simulink model "buckConverterVCM"  (R2024a)
settings: Solver=VariableStepAuto  StartTime=0.0  StopTime=.2  MaxStep=.00001  RelTol=1e-3
model workspace (MAT data in the model file):
  C = Simulink.Parameter
  C.Value = 1e-05
  C.Complexity = 'real'
  C.Dimensions = [1 1]
  C.DataType = 'auto'
  L = Simulink.Parameter
  L.Value = 0.00022
  L.Complexity = 'real'
  L.Dimensions = [1 1]
  L.DataType = 'auto'
  R = Simulink.Parameter
  R.Value = 5
  R.Complexity = 'real'
  R.Dimensions = [1 1]
  R.DataType = 'auto'
  Vin = Simulink.Parameter
  Vin.Value = 48
  Vin.Complexity = 'real'
  Vin.Dimensions = [1 1]
  Vin.DataType = 'auto'
values from neighbouring files (symbols this model uses):
  Fs = 1e5    (= 100000)    [lineToOutputTF.m]
  H = Vref/Vin    (= 0.1)    [lineToOutputTF.m]
  L = 220*10^-6    (= 0.00022)    [lineToOutputTF.m]
  R = Vo/Io    (= 6)    [lineToOutputTF.m]
  R1 = 1e4    (= 10000)    [lineToOutputTF.m]
  R2 = 9e4    (= 90000)    [lineToOutputTF.m]
  Vin = 50    [lineToOutputTF.m]
  Vo = 12    [lineToOutputTF.m]
libraries: spsSeriesRLCBranchLib x5, spsCurrentMeasurementLib x2, spsVoltageMeasurementLib x2, spsControlledVoltageSourceLib x1, spsDiodeLib x1, spsMosfetLib x1, simulink x1, spspowerguiLib x1
settings Model: Creator=User  LastModifiedBy=User
settings DebuggingCC: UnconnectedInputMsg=warning  UnconnectedOutputMsg=warning  UnconnectedLineMsg=warning
settings ModelReferenceCC: EnableRefExpFcnMdlSchedulingChecks=on
settings RTWCC: GPUComputeCapability=3.5  DLArmComputeVersion=19.05

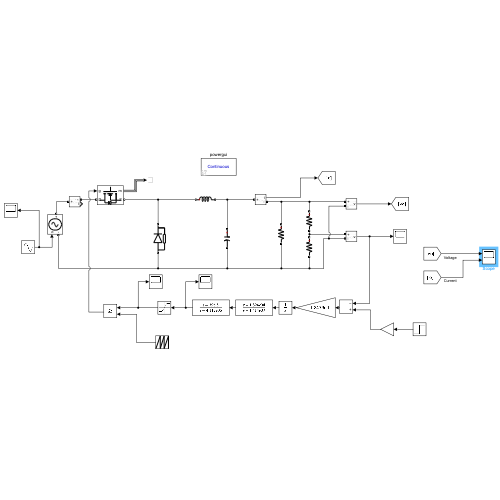
[thumbnail: Simulink's stored preview of the top-level diagram]
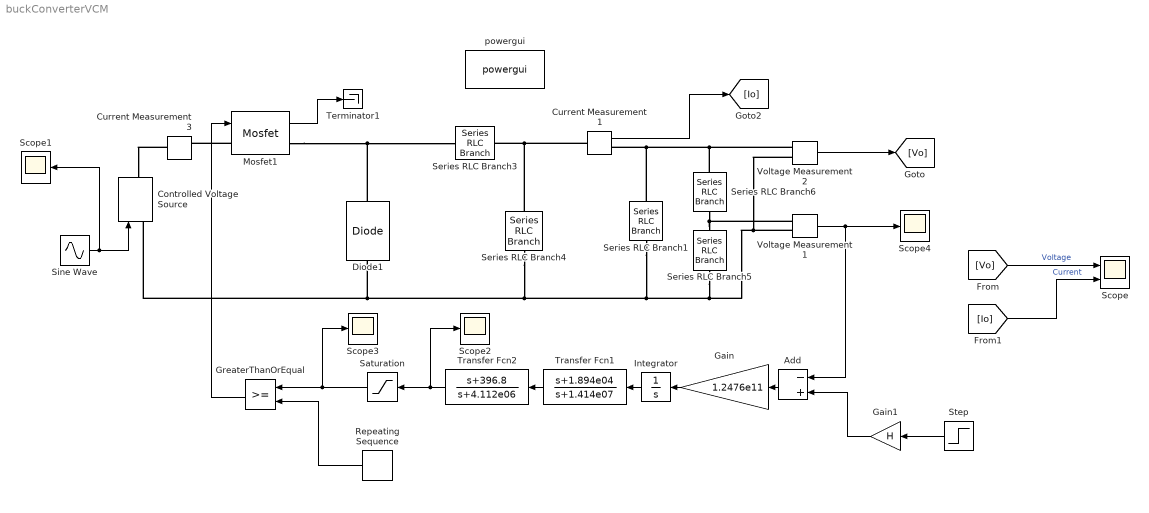
== system buckConverterVCM ==
  Add : Sum  Inputs=-+
  Controlled Voltage Source : spsControlledVoltageSourceLib/Controlled Voltage Source  Initialize=on  Source_Type=AC  Amplitude=0  Phase=0  Frequency=0  Measurements=None
  Current Measurement1 : spsCurrentMeasurementLib/Current Measurement  PhasorSimulation=off  OutputType=Complex  PSBequivalent=0
  Current Measurement3 : spsCurrentMeasurementLib/Current Measurement  PhasorSimulation=off  OutputType=Complex  PSBequivalent=0
  Diode1 : spsDiodeLib/Diode  Ron=0.001  Lon=0  Vf=0.8  IC=0  UseSnubber=0  Rs=500  Cs=250e-9  Measurements=off
  Gain : Gain  Gain=1.2476e11
  Gain1 : Gain  Gain=H
  GreaterThanOrEqual : RelationalOperator  OutDataTypeStr=boolean  RndMeth=Simplest  InputSameDT=off
  Integrator : Integrator
  Mosfet1 : spsMosfetLib/Mosfet  Ron=0.1  Lon=0  Rd=0.01  Vfd=0  IC=0  Rs=1e5  Cs=inf  Measurements=on
  Repeating Sequence : simulink/Sources/Repeating Sequence  rep_seq_t=[0 1]/Fs  rep_seq_y=[0 1]
  Saturation : Saturate  UpperLimit=.9  LowerLimit=.1
  Scope : Scope  NumInputPorts=2
  Scope{1..4} (4 alike) : Scope
  Series RLC Branch1 : spsSeriesRLCBranchLib/Series RLC Branch  LConnTagsString=__new0  RConnTagsString=__new0  BranchType=R  Resistance=R  Inductance=1e-3  SetiL0=off  InitialCurrent=0  Capacitance=1e-6  Setx0=off  InitialVoltage=0  Measurements=None
  Series RLC Branch3 : spsSeriesRLCBranchLib/Series RLC Branch  LConnTagsString=__new0  RConnTagsString=__new0  BranchType=L  Resistance=1  Inductance=L  SetiL0=off  InitialCurrent=0  Capacitance=1e-6  Setx0=off  InitialVoltage=0  Measurements=None
  Series RLC Branch4 : spsSeriesRLCBranchLib/Series RLC Branch  LConnTagsString=__new0  RConnTagsString=__new0  BranchType=C  Resistance=1  Inductance=1e-3  SetiL0=off  InitialCurrent=0  Capacitance=5*10^-4  Setx0=off  InitialVoltage=0  Measurements=None
  Series RLC Branch5 : spsSeriesRLCBranchLib/Series RLC Branch  LConnTagsString=__new0  RConnTagsString=__new0  BranchType=R  Resistance=R1  Inductance=1e-3  SetiL0=off  InitialCurrent=0  Capacitance=1e-6  Setx0=off  InitialVoltage=0  Measurements=None
  Series RLC Branch6 : spsSeriesRLCBranchLib/Series RLC Branch  LConnTagsString=__new0  RConnTagsString=__new0  BranchType=R  Resistance=R2  Inductance=1e-3  SetiL0=off  InitialCurrent=0  Capacitance=1e-6  Setx0=off  InitialVoltage=0  Measurements=None
  Sine Wave : Sin  Amplitude=2  Bias=Vin  Frequency=2*pi*100  SampleTime=0
  Step : Step  Time=0  After=Vo  SampleTime=0
  Terminator1 : Terminator
  Transfer Fcn1 : TransferFcn  Numerator=[1 1.894e04]  Denominator=[1 1.414e07]
  Transfer Fcn2 : TransferFcn  Numerator=[1 396.8]  Denominator=[1 4.112e06]
  Voltage Measurement1 : spsVoltageMeasurementLib/Voltage Measurement  PhasorSimulation=off  OutputType=Complex  PSBequivalent=0
  Voltage Measurement2 : spsVoltageMeasurementLib/Voltage Measurement  PhasorSimulation=off  OutputType=Complex  PSBequivalent=0
  powergui : spspowerguiLib/powergui  Priority=1  SimulationMode=Continuous  SampleTime=50e-6  frequency=60  Iterations=50  frequencyindice=0  Pbase=100e6  ErrMax=1e-4  UnitsV=kV  UnitsW=MW  buscounter=0  FunctionMessages=off  echomessages=off  EnableUseOfTLC=off  CurrentSourceSwitches=off  DisableSnubberDevices=off  DisableRonSwitches=off  DisableVfSwitches=off  DisplayEquations=off  AutomaticDiscreteSolvers=off  SolverType=Tustin/Backward Euler (TBE)  Interpol=off  ExternalGateDelay=off  methode=off  Ts=100  x0status=blocks  SPID=on  SwTol=0  HookPort=off  NonlinearTolerance=1e-4  nMaxIteration=100  ContinueOnMaxIteration=off  RestoreLinks=warning  ResistiveCurrentMeasurement=off  Frange=[0:2:500]  Ylog=off  Xlog=on  ShowGrid=off  save=off  variable=ZData  structure=0  ZoomFFT=off  StartTime=0.0  cycles=1  DisplayStyle=1  fundamental=60  FreqAxis=off  MaxFrequency=1000  frequencyindicesteady=1  RmsSteady=1  display=off
  wires:
  Mosfet1/1 -> Terminator1/1
  Voltage Measurement1/1 -> Scope4/1, Add/1
  Add/1 -> Gain/1
  Transfer Fcn2/1 -> Saturation/1, Scope2/1
  GreaterThanOrEqual/1 -> Mosfet1/1
  Saturation/1 -> GreaterThanOrEqual/1, Scope3/1
  Transfer Fcn1/1 -> Transfer Fcn2/1
  Gain/1 -> Integrator/1
  Integrator/1 -> Transfer Fcn1/1
  Current Measurement1/1 -> [Io]
  Step/1 -> Gain1/1
  Sine Wave/1 -> Scope1/1, Controlled Voltage Source/1
  [Vo] -> Scope/1  "Voltage"
  [Io] -> Scope/2  "Current"
  Gain1/1 -> Add/2
  Voltage Measurement2/1 -> [Vo]
  Repeating Sequence/1 -> GreaterThanOrEqual/2
  connections:
  Series RLC Branch5/RConn1 -- Voltage Measurement2/LConn2 -- Voltage Measurement1/LConn2 -- Series RLC Branch1/RConn1 -- Series RLC Branch4/RConn1 -- Controlled Voltage Source/LConn1 -- Diode1/LConn1
  Diode1/RConn1 -- Series RLC Branch3/LConn1 -- Mosfet1/RConn1
  Current Measurement3/LConn1 -- Controlled Voltage Source/RConn1
  Series RLC Branch4/LConn1 -- Current Measurement1/LConn1 -- Series RLC Branch3/RConn1
  Mosfet1/LConn1 -- Current Measurement3/RConn1
  Series RLC Branch6/RConn1 -- Series RLC Branch5/LConn1 -- Voltage Measurement1/LConn1
  Series RLC Branch6/LConn1 -- Voltage Measurement2/LConn1 -- Current Measurement1/RConn1 -- Series RLC Branch1/LConn1
